simulink library "THBCreator"  (R2013b)
settings: Solver=ode45  StartTime=0.0  StopTime=10.0  RelTol=1e-3
settings Model: Creator=lena.frank  LastModifiedBy=drhf

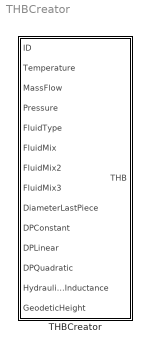
== system THBCreator ==
  THBCreator : Subsystem  InitFcn=load('THB.mat');  mask(THBCreator){Inport_ID=on, Inport_T=on, Inport_mdot=on, Inport_p=on, Inport_type=on, Inport_mix=on, Inport_mix2=on, Inport_mix3=on, Inport_d=on, Inport_c=on, Inport_l=on, Inport_q=on, Inport_LH=on, Inport_H=on, ID=20001, T=20, mdot=0, p=1e5, FluidType=1, FluidMix=0, FluidMix2=0, FluidMix3=0, d=0.02, c=0, l=0, q=0, LH=0, H=0, Annotation_ID=off, Annotation_T=off, Annotation_mdot=off, Annotation_p=off, Annotation_type=off, Annotation_mix=off, Annotation_mix2=off, Annotation_mix3=off, Annotation_d=off, Annotation_c=off, Annotation_l=off, Annotation_q=off, Annotation_LH=off, Annotation_H=off}
      mask prompts: Inport_ID "ID as inport"; Inport_T "temperature as inport"; Inport_mdot "mass flow rate as inport"; Inport_p "pressure as inport"; Inport_type "fluid type as inport"; Inport_mix "fluid mix as inport"; Inport_mix2 "fluid mix2 as inport"; Inport_mix3 "fluid mix3 as inport"; Inport_d "diameter last piece as inport"; Inport_c "constant pressure drop coefficient as inport"; Inport_l "linear pressure drop coefficient as inport"; Inport_q "quadratic pressure drop coefficient as inport"; Inport_LH "hydraulic inductance as inport"; Inport_H "geodetic height as inport"; ID "ID [1]"; T "temperature [°C]"; mdot "mass flow rate [kg/s]"; p "pressure [Pa]"; FluidType "fluid type [enum]"; FluidMix "fluid mix [1]"; FluidMix2 "fluid mix [2]"; FluidMix3 "fluid mix [3]"; d "diameter last piece [m]"; c "constant pressure drop coefficient [Pa]"; l "linear pressure drop coefficient [Pa/(kg/s)]"; q "quadratic pressure drop coefficient [Pa/(kg/s)²]"; LH "hydraulic inductance [1/m]"; H "geodetic height"; Annotation_ID "ID as annotation"; Annotation_T "temperature as annotation"; Annotation_mdot "mass flow rate as annotation"; Annotation_p "pressure as annotation"; Annotation_type "fluid type as annotation"; Annotation_mix "fluid mix as annotation"; Annotation_mix2 "fluid mix2 as annotation"; Annotation_mix3 "fluid mix3 as annotation"; Annotation_d "diameter last piece as annotation"; Annotation_c "constant pressure drop coefficient as annotation"; Annotation_l "linear pressure drop coefficient as annotation"; Annotation_q "quadratic pressure drop coefficient as annotation"; Annotation_LH "hydraulic inductance as annotation"; Annotation_H "geodetic height as annotation"
      mask help: This block creates a THB from input signals.
      mask init:
      | CarnotCallbacks_THBCreator('CreateInports', gcb);
      mask Help:
      | web('THBCreator.html','-helpbrowser'
      | web(fullfile(path_carnot('help'),'THBCreator.html'),'-helpbrowser')
      mask Callback Inport_ID:
      | CarnotCallbacks_THBCreator('CreateMaskVisibilities', gcb);
      | CarnotCallbacks_THBCreator('CreateMaskAnnotations', gcb);
      mask Callback Inport_T:
      | CarnotCallbacks_THBCreator('CreateMaskVisibilities', gcb);
      | CarnotCallbacks_THBCreator('CreateMaskAnnotations', gcb);
      mask Callback Inport_mdot:
      | CarnotCallbacks_THBCreator('CreateMaskVisibilities', gcb);
      | CarnotCallbacks_THBCreator('CreateMaskAnnotations', gcb);
      mask Callback Inport_p:
      | CarnotCallbacks_THBCreator('CreateMaskVisibilities', gcb);
      | CarnotCallbacks_THBCreator('CreateMaskAnnotations', gcb);
      mask Callback Inport_type:
      | CarnotCallbacks_THBCreator('CreateMaskVisibilities', gcb);
      | CarnotCallbacks_THBCreator('CreateMaskAnnotations', gcb);
      mask Callback Inport_mix:
      | CarnotCallbacks_THBCreator('CreateMaskVisibilities', gcb);
      | CarnotCallbacks_THBCreator('CreateMaskAnnotations', gcb);
      mask Callback Inport_mix2:
      | CarnotCallbacks_THBCreator('CreateMaskVisibilities', gcb);
      | CarnotCallbacks_THBCreator('CreateMaskAnnotations', gcb);
      mask Callback Inport_mix3:
      | CarnotCallbacks_THBCreator('CreateMaskVisibilities', gcb);
      | CarnotCallbacks_THBCreator('CreateMaskAnnotations', gcb);
      mask Callback Inport_d:
      | CarnotCallbacks_THBCreator('CreateMaskVisibilities', gcb);
      | CarnotCallbacks_THBCreator('CreateMaskAnnotations', gcb);
      mask Callback Inport_c:
      | CarnotCallbacks_THBCreator('CreateMaskVisibilities', gcb);
      | CarnotCallbacks_THBCreator('CreateMaskAnnotations', gcb);
      mask Callback Inport_l:
      | CarnotCallbacks_THBCreator('CreateMaskVisibilities', gcb);
      | CarnotCallbacks_THBCreator('CreateMaskAnnotations', gcb);
      mask Callback Inport_q:
      | CarnotCallbacks_THBCreator('CreateMaskVisibilities', gcb);
      | CarnotCallbacks_THBCreator('CreateMaskAnnotations', gcb);
      mask Callback Inport_LH:
      | CarnotCallbacks_THBCreator('CreateMaskVisibilities', gcb);
      | CarnotCallbacks_THBCreator('CreateMaskAnnotations', gcb);
      mask Callback Inport_H:
      | CarnotCallbacks_THBCreator('CreateMaskVisibilities', gcb);
      | CarnotCallbacks_THBCreator('CreateMaskAnnotations', gcb);
      mask Callback ID: CarnotCallbacks_THBCreator('CreateMaskAnnotations', gcb);
      mask Callback T: CarnotCallbacks_THBCreator('CreateMaskAnnotations', gcb);
      mask Callback mdot: CarnotCallbacks_THBCreator('CreateMaskAnnotations', gcb);
      mask Callback p: CarnotCallbacks_THBCreator('CreateMaskAnnotations', gcb);
      mask Callback FluidType: CarnotCallbacks_THBCreator('CreateMaskAnnotations', gcb);
      mask Callback FluidMix: CarnotCallbacks_THBCreator('CreateMaskAnnotations', gcb);
      mask Callback FluidMix2: CarnotCallbacks_THBCreator('CreateMaskAnnotations', gcb);
      mask Callback FluidMix3: CarnotCallbacks_THBCreator('CreateMaskAnnotations', gcb);
      mask Callback d: CarnotCallbacks_THBCreator('CreateMaskAnnotations', gcb);
      mask Callback c: CarnotCallbacks_THBCreator('CreateMaskAnnotations', gcb);
      mask Callback l: CarnotCallbacks_THBCreator('CreateMaskAnnotations', gcb);
      mask Callback q: CarnotCallbacks_THBCreator('CreateMaskAnnotations', gcb);
      mask Callback LH: CarnotCallbacks_THBCreator('CreateMaskAnnotations', gcb);
      mask Callback H: CarnotCallbacks_THBCreator('CreateMaskAnnotations', gcb);
      mask Callback Annotation_ID: CarnotCallbacks_THBCreator('CreateMaskAnnotations', gcb);
      mask Callback Annotation_T: CarnotCallbacks_THBCreator('CreateMaskAnnotations', gcb);
      mask Callback Annotation_mdot: CarnotCallbacks_THBCreator('CreateMaskAnnotations', gcb);
      mask Callback Annotation_p: CarnotCallbacks_THBCreator('CreateMaskAnnotations', gcb);
      mask Callback Annotation_type: CarnotCallbacks_THBCreator('CreateMaskAnnotations', gcb);
      mask Callback Annotation_mix: CarnotCallbacks_THBCreator('CreateMaskAnnotations', gcb);
      mask Callback Annotation_mix2: CarnotCallbacks_THBCreator('CreateMaskAnnotations', gcb);
      mask Callback Annotation_mix3: CarnotCallbacks_THBCreator('CreateMaskAnnotations', gcb);
      mask Callback Annotation_d: CarnotCallbacks_THBCreator('CreateMaskAnnotations', gcb);
      mask Callback Annotation_c: CarnotCallbacks_THBCreator('CreateMaskAnnotations', gcb);
      mask Callback Annotation_l: CarnotCallbacks_THBCreator('CreateMaskAnnotations', gcb);
      mask Callback Annotation_q: CarnotCallbacks_THBCreator('CreateMaskAnnotations', gcb);
      mask Callback Annotation_LH: CarnotCallbacks_THBCreator('CreateMaskAnnotations', gcb);
      mask Callback Annotation_H: CarnotCallbacks_THBCreator('CreateMaskAnnotations', gcb);

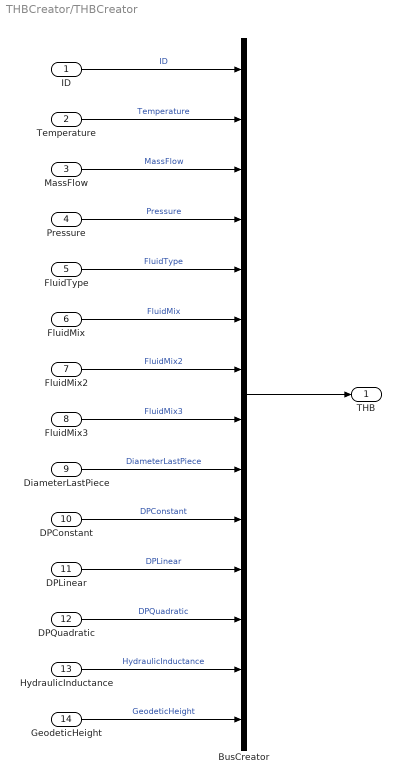
== system THBCreator/THBCreator ==
  ID : Inport
  Temperature : Inport  Port=2
  MassFlow : Inport  Port=3
  Pressure : Inport  Port=4
  FluidType : Inport  Port=5
  FluidMix : Inport  Port=6
  FluidMix2 : Inport  Port=7
  FluidMix3 : Inport  Port=8
  DiameterLastPiece : Inport  Port=9
  DPConstant : Inport  Port=10
  DPLinear : Inport  Port=11
  DPQuadratic : Inport  Port=12
  HydraulicInductance : Inport  Port=13
  GeodeticHeight : Inport  Port=14
  BusCreator : BusCreator  Inputs=14  OutDataTypeStr=Bus: THB
  THB : Outport  OutDataTypeStr=Bus: THB
  wires:
  GeodeticHeight/1 -> BusCreator/14  "GeodeticHeight"
  HydraulicInductance/1 -> BusCreator/13  "HydraulicInductance"
  DPQuadratic/1 -> BusCreator/12  "DPQuadratic"
  DPLinear/1 -> BusCreator/11  "DPLinear"
  DPConstant/1 -> BusCreator/10  "DPConstant"
  DiameterLastPiece/1 -> BusCreator/9  "DiameterLastPiece"
  FluidMix3/1 -> BusCreator/8  "FluidMix3"
  FluidMix2/1 -> BusCreator/7  "FluidMix2"
  FluidMix/1 -> BusCreator/6  "FluidMix"
  FluidType/1 -> BusCreator/5  "FluidType"
  Pressure/1 -> BusCreator/4  "Pressure"
  MassFlow/1 -> BusCreator/3  "MassFlow"
  Temperature/1 -> BusCreator/2  "Temperature"
  ID/1 -> BusCreator/1  "ID"
  BusCreator/1 -> THB/1
